simulink model "wk2_1"  (R2020b)
settings: Solver=VariableStepAuto  StartTime=0.0  StopTime=100  RelTol=1e-3
settings Model: Creator=hp  LastModifiedBy=ASUS

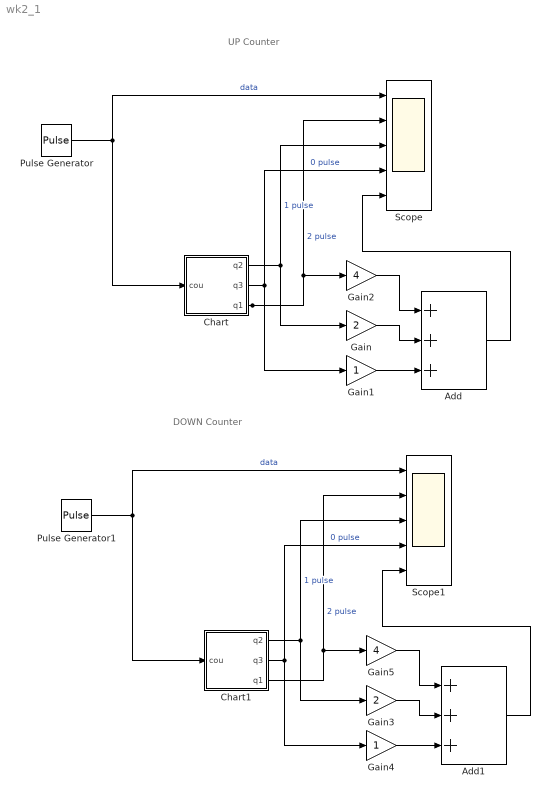
== system wk2_1 ==
  note: UP Counter
  note: DOWN Counter
  Add : Sum  Inputs=+++
  Add1 : Sum  Inputs=+++
  Chart : Stateflow chart  TreatAsAtomicUnit=on
  Chart1 : Stateflow chart  TreatAsAtomicUnit=on
  Gain : Gain  Gain=2
  Gain1 : Gain
  Gain2 : Gain  Gain=4
  Gain3 : Gain  Gain=2
  Gain4 : Gain
  Gain5 : Gain  Gain=4
  Pulse Generator : DiscretePulseGenerator  PulseType=Time based  Period=10  PulseWidth=50
  Pulse Generator1 : DiscretePulseGenerator  PulseType=Time based  Period=10  PulseWidth=50
  Scope : Scope  NumInputPorts=5
  Scope1 : Scope  NumInputPorts=5
  wires:
  Gain/1 -> Add/2
  Gain1/1 -> Add/3
  Chart/1(q2) -> Gain/1, Scope/3  "1 pulse"
  Add/1 -> Scope/5
  Chart/2(q3) -> Scope/4, Gain1/1  "0 pulse"
  Pulse Generator/1 -> Chart/1(cou), Scope/1  "data"
  Gain2/1 -> Add/1
  Chart/3(q1) -> Scope/2, Gain2/1  "2 pulse"
  Gain4/1 -> Add1/3
  Pulse Generator1/1 -> Chart1/1(cou), Scope1/1  "data"
  Add1/1 -> Scope1/5
  Chart1/1(q2) -> Gain3/1, Scope1/3  "1 pulse"
  Chart1/2(q3) -> Scope1/4, Gain4/1  "0 pulse"
  Chart1/3(q1) -> Scope1/2, Gain5/1  "2 pulse"
  Gain5/1 -> Add1/1
  Gain3/1 -> Add1/2

== stateflow chart wk2_1/Chart1 ==
  state a_case5
    entry:
    q1=1;
    q2=0;
    q3=0;
  state a_case1
    entry:
    q1=0;
    q2=0;
    q3=0;
  state a000
    entry:
    q1=0;
    q2=0;
    q3=0;
  state a0004
    entry:
    q1=1;
    q2=0;
    q3=0;
  state a0001
    entry:
    q1=0;
    q2=0;
    q3=1;
  state a_case4
    entry:
    q1=0;
    q2=1;
    q3=1;
  state a_case2
    entry:
    q1=0;
    q2=0;
    q3=1;
  state a0003
    entry:
    q1=0;
    q2=1;
    q3=1;
  state a0002
    entry:
    q1=0;
    q2=1;
    q3=0;
  state a_case3
    entry:
    q1=0;
    q2=1;
    q3=0;
  (default) -> a000
  a000 -> a_case5 : [cou==1]
  a_case1 -> a000 : [cou==0]
  a_case5 -> a0004 : [cou==0]
  a0001 -> a_case1 : [cou==1]
  a0004 -> a_case4 : [cou==1]
  a_case2 -> a0001 : [cou==0]
  a_case4 -> a0003 : [cou==0]
  a0002 -> a_case2 : [cou==1]
  a0003 -> a_case3 : [cou==1]
  a_case3 -> a0002 : [cou==0]
  data: q2 output; q3 output; q1 output; cou input

== stateflow chart wk2_1/Chart ==
  state a_case5
    entry:
    q1=1;
    q2=0;
    q3=0;
  state a_case1
    entry:
    q1=0;
    q2=0;
    q3=0;
  state a000
    entry:
    q1=0;
    q2=0;
    q3=0;
  state a0004
    entry:
    q1=1;
    q2=0;
    q3=0;
  state a0001
    entry:
    q1=0;
    q2=0;
    q3=1;
  state a_case4
    entry:
    q1=0;
    q2=1;
    q3=1;
  state a_case2
    entry:
    q1=0;
    q2=0;
    q3=1;
  state a0003
    entry:
    q1=0;
    q2=1;
    q3=1;
  state a0002
    entry:
    q1=0;
    q2=1;
    q3=0;
  state a_case3
    entry:
    q1=0;
    q2=1;
    q3=0;
  (default) -> a000
  a_case5 -> a000 : [cou==1]
  a000 -> a_case1 : [cou==0]
  a0004 -> a_case5 : [cou==0]
  a_case1 -> a0001 : [cou==1]
  a_case4 -> a0004 : [cou==1]
  a0001 -> a_case2 : [cou==0]
  a0003 -> a_case4 : [cou==0]
  a_case2 -> a0002 : [cou==1]
  a_case3 -> a0003 : [cou==1]
  a0002 -> a_case3 : [cou==0]
  data: q2 output; q3 output; q1 output; cou input
